simulink model "CoditionalStatement"  (R2026a)
settings: Solver=VariableStepAuto
StartFcn:
  | learning.simulink.modelCallbacks.startFunction(gcs);
StopFcn:
  | learning.simulink.modelCallbacks.stopFunction(gcs);
model workspace (MAT data in the model file):
  courseObject.course = 'simulink'
  courseObject.chapter = 4
  courseObject.lesson = 3
  courseObject.section = 1
  courseObject.task = 1
  t_ans = [0; 0.2; 0.20135792079; 0.20135792079; 0.20135792079; 0.40135792079; 0.60135792079; 0.80135792079; 1.00135792079; 1.20135792079; 1.40135792079; 1.60135792079; 1.80135792079; 2.00135792079; 2.20135792079; 2.40135792079; 2.60135792079; 2.80135792079; 2.9402347328; 2.9402347328; 3.1402347328; 3.3402347328; 3.5402347328; 3.7402347328; 3.9402347328; 4.1402347328; 4.3402347328; 4.5402347328; 4.7402347328; 4.9402347328; 5.1402347328; 5.3402347328; 5.5402347328; 5.7402347328; 5.9402347328; 6.1402347328; 6.3402347328; 6.48454322797; 6.48454322797; 6.68454322797; 6.88454322797; 7.08454322797; 7.28454322797; 7.48454322797; 7.68454322797; 7.88454322797; 8.08454322797; 8.28454322797; 8.48454322797; 8.68454322797; 8.88454322797; 9.08454322797; 9.22342003998; 9.22342003998; 9.42342003998; 9.62342003998; 9.82342003998; 10]
  y_ans = [-2; -2; -2; -2; 0.2; 0.390668710763; 0.565762692855; 0.71830150175; 0.842203896502; 0.932530279628; 0.985679623275; 0.999533030834; 0.973538210663; 0.908731494209; 0.80769652075; 0.674461235842; 0.514337309847; 0.333708378393; 0.2; -2; -2; -2; -2; -2; -2; -2; -2; -2; -2; -2; -2; -2; -2; -2; -2; -2; -2; -2; 0.2; 0.390668710764; 0.565762692855; 0.71830150175; 0.842203896502; 0.932530279628; 0.985679623275; 0.999533030834; 0.973538210663; 0.908731494209; 0.80769652075; 0.674461235842; 0.514337309847; 0.333708378393; 0.2; -2; -2; -2; -2; -2]
libraries: signalChecks x1
CloseFcn:
  | learning.simulink.cleanupOnlineTraining;learning.simulink.Application.getInstance().dduxLogMatlabEvent("ModelClosed");
Description:
  | TrainingCourseModel
settings Model: Creator=PC  LastModifiedBy=PC

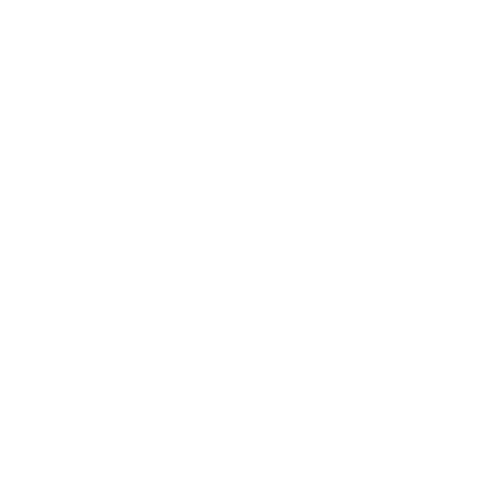
[thumbnail: Simulink's stored preview of the top-level diagram]
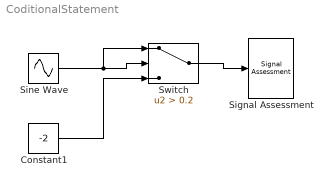
== system CoditionalStatement ==
  Constant1 : Constant  Value=-2
  Signal Assessment : signalChecks/Signal Assessment  signal_type='signal'  t_ans=t_ans  y_ans_upper=y_ans  y_ans_lower=0  range=0.005  rate_type=0  lesson=0  task=3  pass=1
  Sine Wave : Sin  SampleTime=0
  Switch : Switch  Criteria=u2 > Threshold  Threshold=0.2  SaturateOnIntegerOverflow=off  InputSameDT=off
  wires:
  Sine Wave/1 -> Switch/1, Switch/2
  Constant1/1 -> Switch/3
  Switch/1 -> Signal Assessment/1
